simulink model "BLDC_OpenLoop_s32k144"  (Simulink 9.0)
settings: Solver=FixedStepDiscrete  StartTime=0.0  StopTime=10.0  FixedStep=0.1  RelTol=1e-3  EnableMultiTasking=on
model workspace (MAT data in the model file):
  ALIGN_TIME = Simulink.Parameter
  ALIGN_TIME.Value = 20
  ALIGN_TIME.Description = 'number of model fixed-step size steps.'
  ALIGN_TIME.DataType = 'uint16'
  ALIGN_TIME.Min = 0
  ALIGN_TIME.Max = 100
  ALIGN_TIME.Dimensions = [1 1]
  IDC_OVERCURRENT = Simulink.Parameter
  IDC_OVERCURRENT.Value = 4
  IDC_OVERCURRENT.DataType = 'single'
  IDC_OVERCURRENT.Min = 0
  IDC_OVERCURRENT.Max = 16
  IDC_OVERCURRENT.DocUnits = 'A'
  IDC_OVERCURRENT.Dimensions = [1 1]
  V0 = Simulink.Parameter
  V0.Value = 3
  V0.DataType = 'single'
  V0.Min = 0
  V0.Max = 12
  V0.DocUnits = 'V'
  V0.Dimensions = [1 1]
  VDC_OVERVOLTAGE = Simulink.Parameter
  VDC_OVERVOLTAGE.Value = 18
  VDC_OVERVOLTAGE.DataType = 'single'
  VDC_OVERVOLTAGE.Min = 0
  VDC_OVERVOLTAGE.Max = 18
  VDC_OVERVOLTAGE.DocUnits = 'V'
  VDC_OVERVOLTAGE.Dimensions = [1 1]
  VDC_UNDERVOLTAGE = Simulink.Parameter
  VDC_UNDERVOLTAGE.Value = 8
  VDC_UNDERVOLTAGE.DataType = 'single'
  VDC_UNDERVOLTAGE.Min = 0
  VDC_UNDERVOLTAGE.Max = 18
  VDC_UNDERVOLTAGE.DocUnits = 'V'
  VDC_UNDERVOLTAGE.Dimensions = [1 1]
InitFcn:
  | mbd_s32k_consistency_checks(bdroot(gcs));
undefined symbols (not defined in the file): External, LQFP, One, Shot, TRGMUX_PDB_TRIG
libraries: mbd_s32k1xx_ec_toolbox x40, simulink x8, mbd_msd_ec_toolbox x5, ammclib_bam_s32k14x x2
(part 1 of 2)
Description:
  | Open Loop BLDC example for S32K144 and DevKit MotorGD.
  | This Simulink model is designed to work with Linix 45ZWN24-40 Motor and validate
  | that the motor can be rotated with 6-step commutation method. The main scope of
  | the model is to validate the Hall sensors.
  | 
  | FEATURES:
  | - Voltage command is read via SW2 (CW direction) or SW3 (CCW direction)
  | - Read hall sensors in interrupt more for table commutation (used to drive the MOSFETs)
  | 
  | HW SETUP:
  | - Configure S32K144 board supply voltage: J107:2-3(over USB)
  | - Configure J9,J10 and J11 on MotorGD: 2-3 (mode BLDC)
  | - Rotate trimmer resistor R72 (placed Devkit-MotorGD) counter-clockwise at maximum
  | - Connect the motor phases to MotorGD J13 connector
  |   (i.e. Linix 45ZWN24-40: phA-white/phB-blue/phC-green)
  | - Connect the motor hall sensors to MotorGD JP1 connector
  |   (i.e. Linix 45ZWN24-40: Hall_A-white/Hall_B-blue/Hall_C-green)
  | - Power on the MotorGD via J7 connector with 12Vdc
  | - NOTE! Make sure the R168/R166 are placed and R167/R165 are removed
  | 
  | VALIDATION:
  | - After reset or power on, the Green LED shall be ON after ~5sec
  | - If the Vdc is present and SW2 or SW3 is pressed the Blue LED will be ON
  | - In case of a FAULT the Red LED will be ON
  | - The initial voltage command is set to 3V and can be changed from Simulink Model Wrks
  | - Open FreeMASTER project and connect to the target.
  | - Start by pressing the SW2 or SW3 to command the motor to spin in CW or CCW direction
  | - Press the SW2 or SW3 the modify the motor speed or use FreeMASTER UI panel
  | - Voltage and Current protections for Devkit MotorGD are enabled. If fault occurs the
  |   INVERTER is shut down and RED LED is ON
  | 
  | NOTE:
  | - In case of fault (RED LED is ON), the remove fault cause and press RESET button
  | 
  | Copyright (c) 2019 NXP
  | version 3.2.0
settings Model: Creator=NXP MBDT Team  LastModifiedBy=nxf40284  OrderedModelArguments=off
settings DataIOCC: ExternalInput=off  InitialState=off  LimitDataPoints=on  SaveOutput=off  SignalLogging=off  SaveTime=off
settings OptimizationCC: DefaultParameterBehavior=Inlined  UseFloatMulNetSlope=on  DefaultUnderspecifiedDataType=single  UseSpecifiedMinMax=on  EnhancedBackFolding=on  PassReuseOutputArgsAs=Individual arguments  ZeroExternalMemoryAtStartup=off  ZeroInternalMemoryAtStartup=off  NoFixptDivByZeroProtection=on  EfficientFloat2IntCast=on  LifeSpan=auto  OptimizeBlockOrder=speed  DifferentSizesBufferReuse=on
settings DebuggingCC: CheckSSInitialOutputMsg=off  SolverPrmCheckMsg=warning  InheritedTsInSrcMsg=none  MultiTaskDSMMsg=none  SingleTaskRateTransMsg=error  ParameterPrecisionLossMsg=none  ParameterTunabilityLossMsg=error  UnconnectedInputMsg=error  UnconnectedOutputMsg=error  UnconnectedLineMsg=error  AssertControl=DisableAll  AllowSymbolicDim=off  UnknownTsInhSupMsg=error  StateNameClashWarn=warning  ArithmeticOperatorsInVariantConditions=warning
settings HardwareCC: ProdLargestAtomicInteger=Long  ProdLargestAtomicFloat=Double  ProdIntDivRoundTo=Zero  ProdEndianess=LittleEndian  ProdHWDeviceType=ARM Compatible->ARM Cortex
settings ModelReferenceCC: PropagateSignalLabelsOutOfModel=on
settings SFSimCC: MATLABDynamicMemAlloc=off
settings RTWCC: SystemTargetFile=mbd_s32k.tlc  MakeCommand=mbd_s32k_make_rtw COPY_MDLREF_INCLUDES=0  TemplateMakefile=mbd_s32k.tmf  Description=Model Based Design Toolbox S32K1xx Code Generation Target  IncludeHyperlinkInReport=on
settings CodeAppCC: ForceParamTrailComments=on  IgnoreCustomStorageClasses=off  MaxIdLength=64  OperatorAnnotations=on  SimulinkDataObjDesc=on  SFDataObjDesc=on  InsertBlockDesc=on  StateflowObjectComments=off  InternalIdentifier=Classic
settings STFCustomTargetCC: TargetLangStandard=C99 (ISO)  MultiwordLength=256  CombineOutputUpdateFcns=on  ERTCustomFileBanners=on  SupportContinuousTime=off  SupportNonInlinedSFcns=off  RemoveResetFunc=on  MATLABClassNameForMDSCustomization=Simulink.SoftwareTarget.ERTCustomization  GRTInterface=off  SystemTargetFile=mbd_s32k.tlc
settings ERTTargetCC: TargetLangStandard=C99 (ISO)  ParMdlRefBuildCompliant=off  CompOptLevelCompliant=off  ConcurrentExecutionCompliant=off  ModelStepFunctionPrototypeControlCompliant=off  CPPClassGenCompliant=off  UseToolchainInfoCompliant=off  InlinedParameterPlacement=NonHierarchical  ERTSrcFileBannerTemplate=mbd_ert_code_template.cgt  ERTHdrFileBannerTemplate=mbd_ert_code_template.cgt  ERTDataSrcFileTemplate=mbd_ert_code_template.cgt  ERTDataHdrFileTemplate=mbd_ert_code_template.cgt  ERTCustomFileTemplate=example_file_process.tlc

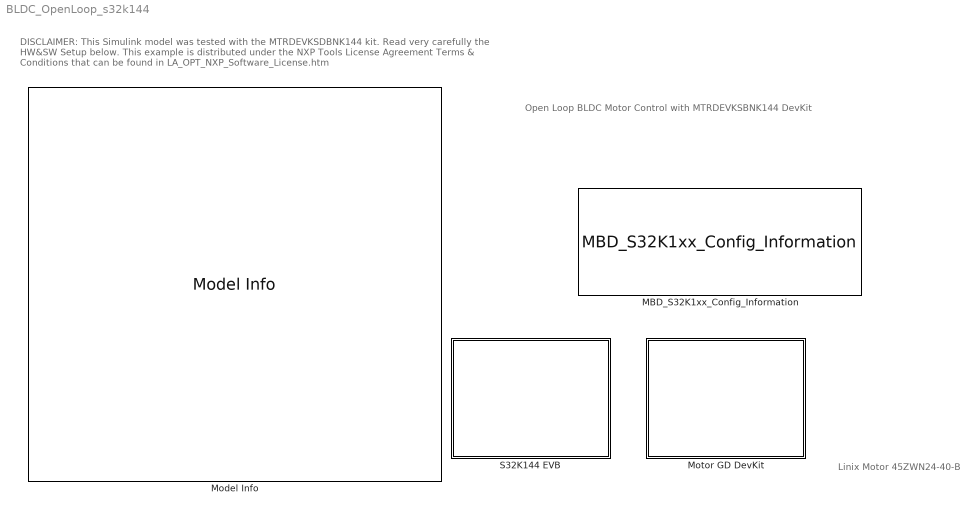
== system BLDC_OpenLoop_s32k144 ==
  note: Linix Motor 45ZWN24-40-B
  note: Open Loop BLDC Motor Control
      | with MTRDEVKSBNK144 DevKit
  note: DISCLAIMER: This Simulink model was tested with the MTRDEVKSDBNK144 kit. Read very carefully the HW&SW Setup below.
      | This example is distributed under the NXP Tools License Agreement Terms & Conditions that can be found in LA_OPT_NXP_Software_License.htm
  MBD_S32K1xx_Config_Information : mbd_s32k1xx_ec_toolbox/MBD_S32K1xx_Config_Information  mbdt_ver=0  disp_str=|  config_params=[]  mcu_target_name=S32K144  mcu_target_package=64-LQFP  mcu_target_sram_size=64KB  mcu_system_clock_freq=80  mcu_xtal_freq=External 8  mcu_steptick_timer=LPIT Channel 0  mcu_steptick_prio=10  ds_import_enable=on  target_compiler=GCC  target_memory=FLASH  gcc_target_compile_opts=-mcpu=cortex-m4 -mthumb -mfloat-abi=hard -mfpu=fpv4-sp-d16 -O1 -g -gstrict-dwarf  gcc_target_assemble_opts=-mcpu=cortex-m4 -mthumb -mfloat-abi=hard -mfpu=fpv4-sp-d16 -g  gcc_target_link_opts=-mcpu=cortex-m4 -mthumb -mfloat-abi=hard -mfpu=fpv4-sp-d16  gcc_target_default_lcf=on  gcc_target_user_lcf=S32K144_64_flash.ld  ghs_target_compile_opts=-cpu=cortexm4f -thumb -fpu=vfpv4_d16 -fsingle -Ogeneral -Wundef -Wimplicit-int -Wshadow -Wtrigraphs --no_commons --gnu_asm -gnu99 -gdwarf-2 -G  ghs_target_assemble_opts=-cpu=cortexm4f -fpu=vfpv4_d16  ghs_target_link_opts=-cpu=cortexm4f -thumb -fpu=vfpv4_d16  ghs_target_default_lcf=on  ghs_target_user_lcf=S32K144_64_flash.ld  iar_target_compile_opts=--cpu=Cortex-M4F --thumb --fpu=VFPv4_sp -Ol -e --debug --dlib_config normal  iar_target_assemble_opts=--cpu Cortex-M4F --thumb --fpu VFPv4_sp  iar_target_link_opts=--no_exceptions --vfe --inline  iar_target_default_lcf=on  iar_target_user_lcf=S32K144_64_flash.icf  pil_download_enable=off  rbl_download_enable=on  rbl_start_delay=5000  rbl_download_interface=OpenSDA  rbl_restart_request=off  rbl_com_port=Custom  rbl_com_port_custom=COM1  pil_download_rate=57600  pil_opensda_drive=Custom  pil_opensda_drive_custom=D  pil_uart_instance=1  pil_uart_rx=PTC6: [LPUART1_RX | Receive]  pil_uart_tx=PTC7: [LPUART1_TX | Transmit]  FTM_PWM_PcrCheckEnDis=on  FTM_Input_Edge_Inputs_PcrCheckEnDis=on  FTM_Dual_Edge_Inputs_PcrCheckEnDis=on  FTM_Quadrature_Inputs_PcrCheckEnDis=on  FTM_Hall_Sensor_Inputs_PcrCheckEnDis=on  LPTMR_PcrCheckEnDis=on  PIT_PcrCheckEnDis=on  RTC_PcrCheckEnDis=on  FlexCAN_PcrCheckEnDis=on  LIN_PcrCheckEnDis=on  FlexIO_PcrCheckEnDis=on  LPI2C_PcrCheckEnDis=on  LPSPI_PcrCheckEnDis=on  LPUART_PcrCheckEnDis=on  CMP_PcrCheckEnDis=on  GPIO_OutputPcrCheckEnDis=on  GPIO_InputPcrCheckEnDis=on  SBC_PcrCheckEnDis=on  AMMCLIB_PcrCheckEnDis=on  FM_PcrCheckEnDis=on  Profile_PcrCheckEnDis=on  ConfigParams_PcrCheckEnDis=on  ModelRef_PcrCheckEnDis=on  PDB0_PcrCheckEnDis=on  CSEc_PcrCheckEnDis=on  eDMA_PcrCheckEnDis=on  ADC_PcrCheckEnDis=on  WDOG_PcrCheckEnDis=on
      | Target : S32K144-64KB_SRAM
      | Package : 100-pin
      | System clock : 80 MHz
      | XTAL clock : External 8 MHz
      | Compiler : IAR
      | Target Type : FLASH
      | Download Code after build : off
      | Step Tick Interrupt Priority : 15
  Model Info : simulink/Model-Wide Utilities/Model Info  Frame=off  DisplayStringWithTags=|  HorizontalTextAlignment=Left  LeftAlignmentValue=0.02
      | Model Name: %<ModelName>
      | 
      | Description: %<Description>
  Motor GD DevKit : Subsystem
      mask Display: image('MotorGD.PNG');
  S32K144 EVB : Subsystem
      mask Display: image('S32K.PNG');

== system BLDC_OpenLoop_s32k144/Motor GD DevKit ==

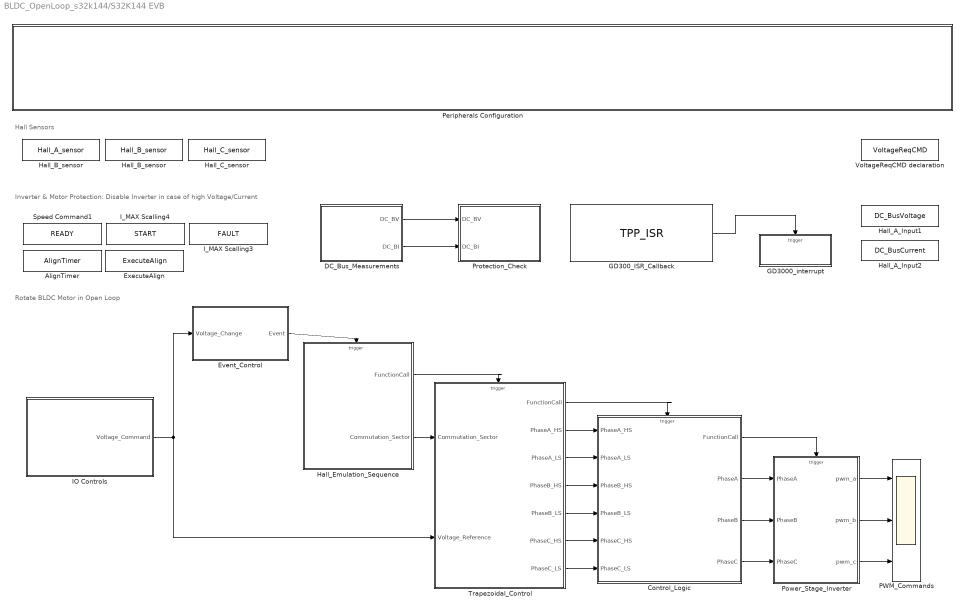
== system BLDC_OpenLoop_s32k144/S32K144 EVB ==
  note: Rotate BLDC Motor in Open Loop
  note: Inverter & Motor Protection: Disable Inverter in case of high Voltage/Current
  note: Hall Sensors
  AlignTimer : DataStoreMemory  DataStoreName=AlignTimer  ReadBeforeWriteMsg=warning  WriteAfterWriteMsg=warning  WriteAfterReadMsg=warning  ShowAdditionalParam=off  OutDataTypeStr=uint16
  Control_Logic : Subsystem
  DC_Bus_Measurements : Subsystem
  Event_Control : Subsystem  TreatAsAtomicUnit=on
      settings: RTWFcnNameOpts=Use subsystem name  RTWFileNameOpts=Use subsystem name
  ExecuteAlign : DataStoreMemory  DataStoreName=ExecuteAlign  ReadBeforeWriteMsg=warning  WriteAfterWriteMsg=warning  WriteAfterReadMsg=warning  InitialValue=1  ShowAdditionalParam=off  OutDataTypeStr=boolean
  GD3000_interrupt : Subsystem  TreatAsAtomicUnit=on
  "GD300_ISR_Callback " : mbd_msd_ec_toolbox/TPP/TPP_ISR  tppInstance=0
  Hall_A_Input1 : DataStoreMemory  DataStoreName=DC_BusVoltage  ReadBeforeWriteMsg=warning  WriteAfterWriteMsg=warning  WriteAfterReadMsg=warning  ShowAdditionalParam=off  OutDataTypeStr=single
  Hall_A_Input2 : DataStoreMemory  DataStoreName=DC_BusCurrent  ReadBeforeWriteMsg=warning  WriteAfterWriteMsg=warning  WriteAfterReadMsg=warning  ShowAdditionalParam=off  OutDataTypeStr=single
  Hall_B_sensor : DataStoreMemory  DataStoreName=Hall_A_sensor  ReadBeforeWriteMsg=warning  WriteAfterWriteMsg=warning  WriteAfterReadMsg=warning  ShowAdditionalParam=off  OutDataTypeStr=boolean
  "Hall_B_sensor " : DataStoreMemory  DataStoreName=Hall_B_sensor  ReadBeforeWriteMsg=warning  WriteAfterWriteMsg=warning  WriteAfterReadMsg=warning  ShowAdditionalParam=off  OutDataTypeStr=boolean
  "Hall_C_sensor " : DataStoreMemory  DataStoreName=Hall_C_sensor  ReadBeforeWriteMsg=warning  WriteAfterWriteMsg=warning  WriteAfterReadMsg=warning  ShowAdditionalParam=off  OutDataTypeStr=boolean
  Hall_Emulation_Sequence : Subsystem
      settings: PropExecContextOutsideSubsystem=on  RTWSystemCode=Nonreusable function  RTWFileNameOpts=Use subsystem name
  "IO Controls " : Subsystem
  I_MAX Scalling3 : DataStoreMemory  DataStoreName=FAULT  ReadBeforeWriteMsg=warning  WriteAfterWriteMsg=warning  WriteAfterReadMsg=warning  ShowAdditionalParam=off  OutDataTypeStr=boolean
  I_MAX Scalling4 : DataStoreMemory  DataStoreName=START  ReadBeforeWriteMsg=warning  WriteAfterWriteMsg=warning  WriteAfterReadMsg=warning  ShowAdditionalParam=off  OutDataTypeStr=boolean
  PWM_Commands : Scope  NumInputPorts=3
  Peripherals Configuration : Subsystem  Priority=1
  Power_Stage_Inverter : Subsystem  TreatAsAtomicUnit=on
      settings: RTWSystemCode=Nonreusable function
  Protection_Check : Subsystem
  Speed Command1 : DataStoreMemory  DataStoreName=READY  ReadBeforeWriteMsg=warning  WriteAfterWriteMsg=warning  WriteAfterReadMsg=warning  ShowAdditionalParam=off  OutMin=0  OutMax=1  OutDataTypeStr=boolean
  Trapezoidal_Control : Subsystem
      settings: RTWSystemCode=Nonreusable function  RTWFcnNameOpts=Use subsystem name
  VoltageReqCMD declaration : DataStoreMemory  Priority=0  DataStoreName=VoltageReqCMD  ReadBeforeWriteMsg=warning  WriteAfterWriteMsg=warning  WriteAfterReadMsg=warning  ShowAdditionalParam=off  OutMin=-12  OutMax=12  OutDataTypeStr=single
  wires:
  Trapezoidal_Control/5(PhaseB_LS) -> Control_Logic/4(PhaseB_LS)
  Trapezoidal_Control/1(FunctionCall) -> Control_Logic/Trigger
  Control_Logic/3(PhaseB) -> Power_Stage_Inverter/2(PhaseB)
  Control_Logic/4(PhaseC) -> Power_Stage_Inverter/3(PhaseC)
  Control_Logic/2(PhaseA) -> Power_Stage_Inverter/1(PhaseA)
  Trapezoidal_Control/6(PhaseC_HS) -> Control_Logic/5(PhaseC_HS)
  Trapezoidal_Control/3(PhaseA_LS) -> Control_Logic/2(PhaseA_LS)
  Control_Logic/1(FunctionCall) -> Power_Stage_Inverter/Trigger
  Trapezoidal_Control/2(PhaseA_HS) -> Control_Logic/1(PhaseA_HS)
  Trapezoidal_Control/7(PhaseC_LS) -> Control_Logic/6(PhaseC_LS)
  Trapezoidal_Control/4(PhaseB_HS) -> Control_Logic/3(PhaseB_HS)
  Power_Stage_Inverter/1(pwm_a) -> PWM_Commands/1
  Power_Stage_Inverter/2(pwm_b) -> PWM_Commands/2
  Power_Stage_Inverter/3(pwm_c) -> PWM_Commands/3
  Event_Control/1(Event) -> Hall_Emulation_Sequence/Trigger
  Hall_Emulation_Sequence/1(FunctionCall) -> Trapezoidal_Control/Trigger
  Hall_Emulation_Sequence/2(Commutation_Sector) -> Trapezoidal_Control/1(Commutation_Sector)
  "IO Controls "/1(Voltage_Command) -> Event_Control/1(Voltage_Change), Trapezoidal_Control/2(Voltage_Reference)
  DC_Bus_Measurements/1(DC_BV) -> Protection_Check/1(DC_BV)
  DC_Bus_Measurements/2(DC_BI) -> Protection_Check/2(DC_BI)
  "GD300_ISR_Callback "/1 -> GD3000_interrupt/Trigger

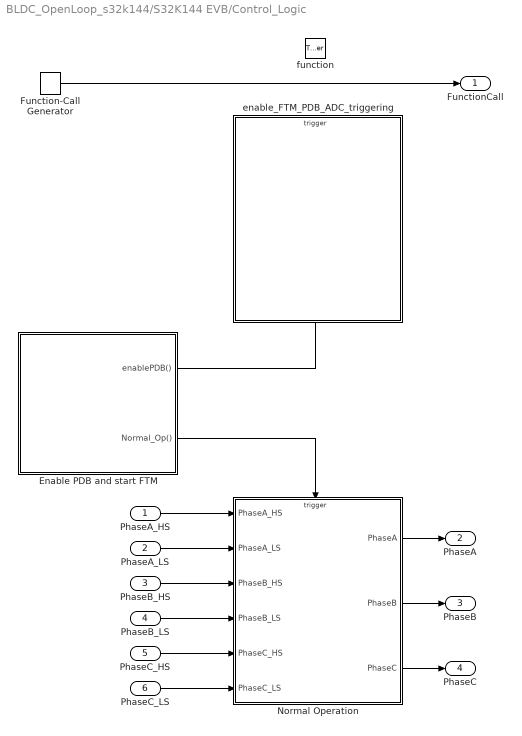
== system BLDC_OpenLoop_s32k144/S32K144 EVB/Control_Logic ==
  PhaseA_HS : Inport
  PhaseA_LS : Inport  Port=2
  PhaseB_HS : Inport  Port=3
  PhaseB_LS : Inport  Port=4
  PhaseC_HS : Inport  Port=5
  PhaseC_LS : Inport  Port=6
  function : TriggerPort  TriggerType=function-call  VariantControl=(inherit)
  Enable PDB and start FTM : Stateflow chart  TreatAsAtomicUnit=on
  Function-Call Generator : simulink/Ports & Subsystems/Function-Call Generator  sample_time=-1  numberOfIterations=1
  Normal Operation : Subsystem  TreatAsAtomicUnit=on
  enable_FTM_PDB_ADC_triggering : Subsystem  TreatAsAtomicUnit=on
      settings: RTWSystemCode=Inline
  FunctionCall : Outport
  PhaseA : Outport  Port=2
  PhaseB : Outport  Port=3
  PhaseC : Outport  Port=4
  wires:
  Enable PDB and start FTM/2(Normal_Op()) -> Normal Operation/Trigger
  Enable PDB and start FTM/1(enablePDB()) -> enable_FTM_PDB_ADC_triggering/Trigger
  Function-Call Generator/1 -> FunctionCall/1
  PhaseB_HS/1 -> Normal Operation/3(PhaseB_HS)
  PhaseB_LS/1 -> Normal Operation/4(PhaseB_LS)
  PhaseA_LS/1 -> Normal Operation/2(PhaseA_LS)
  PhaseC_HS/1 -> Normal Operation/5(PhaseC_HS)
  PhaseA_HS/1 -> Normal Operation/1(PhaseA_HS)
  PhaseC_LS/1 -> Normal Operation/6(PhaseC_LS)
  Normal Operation/2(PhaseB) -> PhaseB/1
  Normal Operation/3(PhaseC) -> PhaseC/1
  Normal Operation/1(PhaseA) -> PhaseA/1

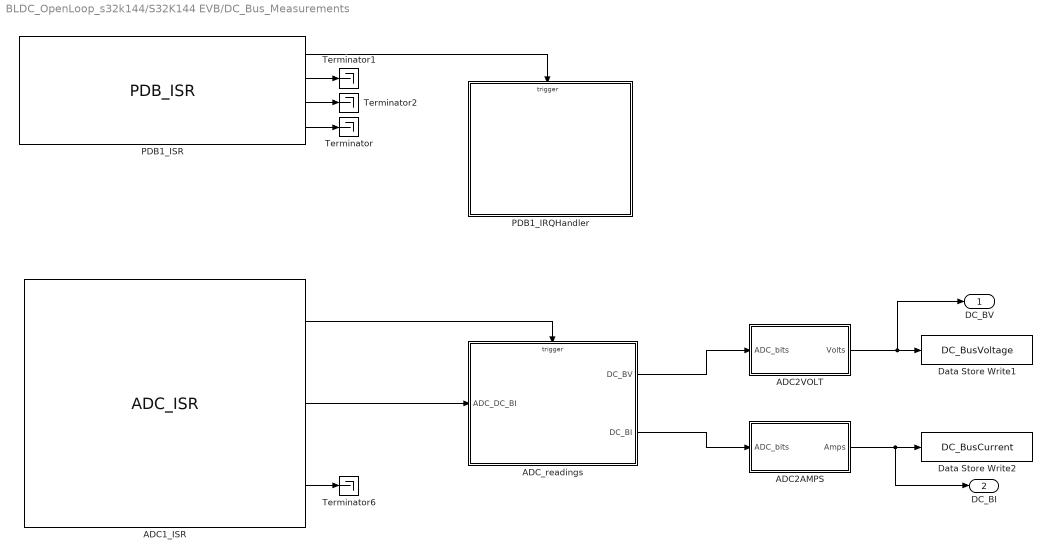
== system BLDC_OpenLoop_s32k144/S32K144 EVB/DC_Bus_Measurements ==
  ADC1_ISR : mbd_s32k1xx_ec_toolbox/Motor Control Blocks/ADC Blocks/ADC_ISR  instance=1  pri=1  sc1n=B
  ADC2AMPS : Subsystem
  ADC2VOLT : Subsystem
  ADC_readings : Subsystem  TreatAsAtomicUnit=on
      settings: RTWSystemCode=Nonreusable function
  Data Store Write1 : DataStoreWrite  DataStoreName=DC_BusVoltage
  Data Store Write2 : DataStoreWrite  DataStoreName=DC_BusCurrent
  PDB1_IRQHandler : Subsystem  TreatAsAtomicUnit=on
      settings: RTWSystemCode=Nonreusable function
  PDB1_ISR : mbd_s32k1xx_ec_toolbox/Motor Control Blocks/PDB Blocks/PDB_ISR  pdbModule=1  prioInterrupt=2  regScPdbie=on  regScPdbeie=off  regIdlyIdly=4999
  Terminator{,1..2,6} (4 alike) : Terminator
  DC_BV : Outport
  DC_BI : Outport  Port=2
  wires:
  ADC2VOLT/1(Volts) -> DC_BV/1, Data Store Write1/1
  ADC_readings/1(DC_BV) -> ADC2VOLT/1(ADC_bits)
  ADC2AMPS/1(Amps) -> DC_BI/1, Data Store Write2/1
  ADC_readings/2(DC_BI) -> ADC2AMPS/1(ADC_bits)
  PDB1_ISR/1 -> PDB1_IRQHandler/Trigger
  PDB1_ISR/4 -> Terminator/1
  PDB1_ISR/2 -> Terminator1/1
  PDB1_ISR/3 -> Terminator2/1
  ADC1_ISR/1 -> ADC_readings/Trigger
  ADC1_ISR/3 -> Terminator6/1
  ADC1_ISR/2 -> ADC_readings/1(ADC_DC_BI)

== system BLDC_OpenLoop_s32k144/S32K144 EVB/Event_Control ==
  Voltage_Change : Inport
  ControlEventLogic : Subsystem  Priority=3
  ControlPollingLogic : Stateflow chart  Priority=2  TreatAsAtomicUnit=on
  HallSensorInit : Subsystem
      settings: RTWFcnNameOpts=Use subsystem name  RTWFileNameOpts=Use subsystem name
  Init : Stateflow chart  Priority=1  TreatAsAtomicUnit=on
  Mux1 : Mux  Inputs=3
  Event : Outport
  wires:
  Mux1/1 -> Event/1
  Voltage_Change/1 -> ControlPollingLogic/1(VoltageChange)
  Init/1(Init()) -> HallSensorInit/Trigger
  ControlEventLogic/1(HallStateChange) -> Mux1/3
  ControlPollingLogic/1(Trigger()) -> Mux1/2
  HallSensorInit/1(Call) -> Mux1/1

== system BLDC_OpenLoop_s32k144/S32K144 EVB/GD3000_interrupt ==
  function : TriggerPort  TriggerType=function-call  VariantControl=Variant
  FAULT_write : DataStoreWrite  DataStoreName=FAULT
  FTM_PWM_Disable_Enable : mbd_s32k1xx_ec_toolbox/Motor Control Blocks/FTM Blocks/FTM_PWM_Disable_Enable  ftmModule=3  action=Disable
  NOK : Constant  OutDataTypeStr=boolean
  TPP_Functional_Mode : mbd_msd_ec_toolbox/TPP/TPP_Functional_Mode  tppInstance=0  action=Sleep
  wires:
  NOK/1 -> FAULT_write/1

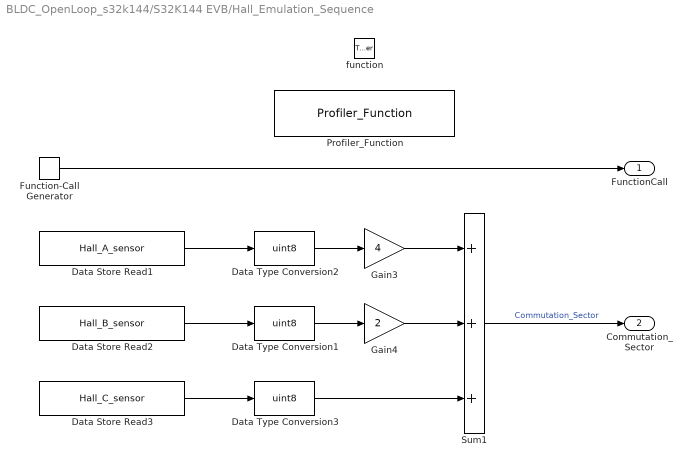
== system BLDC_OpenLoop_s32k144/S32K144 EVB/Hall_Emulation_Sequence ==
  function : TriggerPort  TriggerType=function-call  VariantControl=Variant
  Data Store Read1 : DataStoreRead  DataStoreName=Hall_A_sensor
  Data Store Read2 : DataStoreRead  DataStoreName=Hall_B_sensor
  Data Store Read3 : DataStoreRead  DataStoreName=Hall_C_sensor
  Data Type Conversion1 : DataTypeConversion  OutDataTypeStr=uint8
  Data Type Conversion2 : DataTypeConversion  OutDataTypeStr=uint8
  Data Type Conversion3 : DataTypeConversion  OutDataTypeStr=uint8
  Function-Call Generator : simulink/Ports & Subsystems/Function-Call Generator  sample_time=-1  numberOfIterations=1
  Gain3 : Gain  Gain=4  OutDataTypeStr=uint8  ParamDataTypeStr=Inherit: Same as input
  Gain4 : Gain  Gain=2  OutDataTypeStr=uint8  ParamDataTypeStr=Inherit: Same as input
  Profiler_Function : mbd_s32k1xx_ec_toolbox/Utility Blocks/Profiler_Function  profile_indx=0
  Sum1 : Sum  Inputs=+++  AccumDataTypeStr=uint8
  FunctionCall : Outport
  Commutation_Sector : Outport  Port=2  OutDataTypeStr=uint8
  wires:
  Function-Call Generator/1 -> FunctionCall/1
  Gain3/1 -> Sum1/1
  Gain4/1 -> Sum1/2
  Data Type Conversion2/1 -> Gain3/1
  Data Type Conversion1/1 -> Gain4/1
  Data Type Conversion3/1 -> Sum1/3
  Data Store Read1/1 -> Data Type Conversion2/1
  Data Store Read2/1 -> Data Type Conversion1/1
  Data Store Read3/1 -> Data Type Conversion3/1
  Sum1/1 -> Commutation_Sector/1  "Commutation_Sector"

== system BLDC_OpenLoop_s32k144/S32K144 EVB/IO Controls  ==
  note: RUN STATE
  note: SYSTEM STATE
  If Action Subsystem : Subsystem  TreatAsAtomicUnit=on
  If1 : If  IfExpression=(u1 == 1)  ShowElse=off
  If2 : If  IfExpression=(u1 == 1)  ShowElse=off
  SpeedCmd1 : DataStoreRead  DataStoreName=START
  SpeedCmd2 : DataStoreRead  DataStoreName=FAULT
  SpeedCmd3 : DataStoreRead  DataStoreName=START
  SpeedCmd4 : DataStoreRead  DataStoreName=READY
  Subsystem : Subsystem
  Voltage_Command : Outport
  wires:
  SpeedCmd1/1 -> If1/1
  If1/1 -> If Action Subsystem/Action
  If Action Subsystem/1(Voltage_Command) -> Voltage_Command/1
  SpeedCmd3/1 -> Subsystem/1(START)
  SpeedCmd2/1 -> Subsystem/2(FAULT)
  SpeedCmd4/1 -> If2/1
  If2/1 -> Subsystem/Action

== system BLDC_OpenLoop_s32k144/S32K144 EVB/Peripherals Configuration ==
  ADC1_IRQ : mbd_s32k1xx_ec_toolbox/Motor Control Blocks/ADC Blocks/ADC_Start  Priority=3  instance=1  adc_r=B  adc_chan=PTD4: [ADC1_SE6 | ADC Single Ended Input]  aien=on  mcuTargetUpdate=on
  ADC_Config : mbd_s32k1xx_ec_toolbox/Motor Control Blocks/ADC Blocks/ADC_Config  Priority=2  instance=1  mode=12-bit conversion  smplts=2  adiclk=alternate clock 1  adiv=input clock  show_adv_opts=on  pretrgsel=PDB pre-trigger  swpretrg=Disabled  adtrg=hardware  trgsel=PDB output  refsel=Vrefh and Vrefl  supply_monitoring=off  acfe=off  acfgt=off  acren=off  cv1=0  cv2=0  adco=off  avge=off  avgs=16 samples
  Digital_Input_ISR_Enable_HALL_A : mbd_s32k1xx_ec_toolbox/GPIO Blocks/Digital_Input_ISR_Enable_Disable  gpio_pin=PTD11: [PTD11 | Port D I/O]  irqc=on either-edge
  Digital_Input_ISR_Enable_HALL_B : mbd_s32k1xx_ec_toolbox/GPIO Blocks/Digital_Input_ISR_Enable_Disable  gpio_pin=PTD10: [PTD10 | Port D I/O]  irqc=on either-edge
  Digital_Input_ISR_Enable_HALL_C : mbd_s32k1xx_ec_toolbox/GPIO Blocks/Digital_Input_ISR_Enable_Disable  gpio_pin=PTA1: [PTA1 | Port A I/O]  irqc=on either-edge
  FreeMaster_Config : mbd_s32k1xx_ec_toolbox/Utility Blocks/FreeMaster_Config  interface=LPUART1  baudrate=115200  rxd=PTC6: [LPUART1_RX | Receive]  txd=PTC7: [LPUART1_TX | Transmit]  mode=Short Interrupt  isr_prio=5  show_adv_opts=on  use_scope=on  max_scope_vars=8  use_recorder=on  max_rec_vars=8  rec_buff_size=2048  rec_timebase=1 milliseconds  comm_buffer_size_auto=on  comm_buffer_size=255  comm_rqueue_size_default=on  comm_rqueue_size=32
  GD3000_Config : mbd_msd_ec_toolbox/TPP/TPP_Config  Priority=1  tppInstance=0  desatMode=on  fullonMode=off  lockMode=off  overtempEvent=on  phaseEvent=off  desatEvent=off  framingEvent=on  vlsEvent=on  writeErrEvent=on  overcurrentEvent=on  resetEvent=on  mcuTppIntEn=off  prioInt=15  tppDeadtime=500  initTppNow=on  tppSpiInst=0  tppPwmModule=Please add FTM block to workspace  tppPair0_1=on  tppPair2_3=on  tppPair4_5=on  tppPair6_7=off  tppFirstChHS=on  tppEn1Pin=PTA2: [PTA2 | Port A I/O]  tppEn2Pin=PTA2: [PTA2 | Port A I/O]  tppRstPin=PTA3: [PTA3 | Port A I/O]  tppCsPin=PTB5: [PTB5 | Port B I/O]  tppIntPin=PTE10: [PTE10 | Port E I/O]
  "LPSPI_Config " : mbd_s32k1xx_ec_toolbox/Communication Blocks/SPI Blocks/LPSPI_Config   InstanceNumber=0  Role=Master  BaudRate=2000000  ShowAdvanced=on  sin=PTB3: [LPSPI0_SIN | LPSPI Serial Data Input]  sout=PTB4: [LPSPI0_SOUT | LPSPI Serial Data Output]  sck=PTB2: [LPSPI0_SCK | LPSPI Serial Clock I/O]  pcs0=None  pcs1=PTB5: [LPSPI0_PCS1 | Peripheral Chip Select 1]  pcs2=None  pcs3=None  CPHA=1  CPOL=0  BitOrder=MSB first  TransferSize=8  WhichPCS=0  PCSPol=ActiveLow  ContinuousTransfer=off
  PDB_Config : mbd_s32k1xx_ec_toolbox/Motor Control Blocks/PDB Blocks/PDB_Config  Priority=1  pdbModule=1  regScCont=One-Shot  regScTrgsel=External (TRGMUX_PDB_TRIG)  trgMuxSel=FTM3 Initialize Trigger  trgMuxSelPin=PTB5: [TRGMUX_IN0 | Trigger Mux Input]  regModModulus=5000  regScPrescaler=1  regScMult=1  regPoenPoen0=off  regPo0DlyDly1=0  regPo0DlyDly2=1000  enable_pdb_init=off  show_adv_opts=on  regCh0C1En0=on  regCh0C1En1=on  regCh0C1En2=off  regCh0C1En3=off  regCh0C1En4=off  regCh0C1En5=off  regCh0C1En6=off  regCh0C1En7=off  regCh0C1Bb0=off  regCh0C1Bb1=off  regCh0C1Bb2=off  regCh0C1Bb3=off  regCh0C1Bb4=off  regCh0C1Bb5=off  regCh0C1Bb6=off  regCh0C1Bb7=off  regCh0C1Tos0=Pre-trigger is in delay mode  regCh0C1Tos1=Pre-trigger is in delay mode  regCh0C1Tos2=Pre-trigger is in delay mode  regCh0C1Tos3=Pre-trigger is in delay mode  regCh0C1Tos4=Pre-trigger is in delay mode  regCh0C1Tos5=Pre-trigger is in delay mode  regCh0C1Tos6=Pre-trigger is in delay mode  regCh0C1Tos7=Pre-trigger is in delay mode  regCh0DlyDly0=0  regCh0DlyDly1=200  regCh0DlyDly2=0  regCh0DlyDly3=0  regCh0DlyDly4=0  regCh0DlyDly5=0  regCh0DlyDly6=0  regCh0DlyDly7=0  regCh1C1En0=off  regCh1C1En1=off  regCh1C1En2=off  regCh1C1En3=off  regCh1C1En4=off  regCh1C1En5=off  regCh1C1En6=off  regCh1C1En7=off  regCh1C1Bb0=off  regCh1C1Bb1=off  regCh1C1Bb2=off  regCh1C1Bb3=off  regCh1C1Bb4=off  regCh1C1Bb5=off  regCh1C1Bb6=off  regCh1C1Bb7=off  regCh1C1Tos0=Pre-trigger is in delay mode  regCh1C1Tos1=Pre-trigger is in delay mode  regCh1C1Tos2=Pre-trigger is in delay mode  regCh1C1Tos3=Pre-trigger is in delay mode  regCh1C1Tos4=Pre-trigger is in delay mode  regCh1C1Tos5=Pre-trigger is in delay mode  regCh1C1Tos6=Pre-trigger is in delay mode  regCh1C1Tos7=Pre-trigger is in delay mode  regCh1DlyDly0=100  regCh1DlyDly1=200  regCh1DlyDly2=300  regCh1DlyDly3=400  regCh1DlyDly4=500  regCh1DlyDly5=600  regCh1DlyDly6=700  regCh1DlyDly7=800

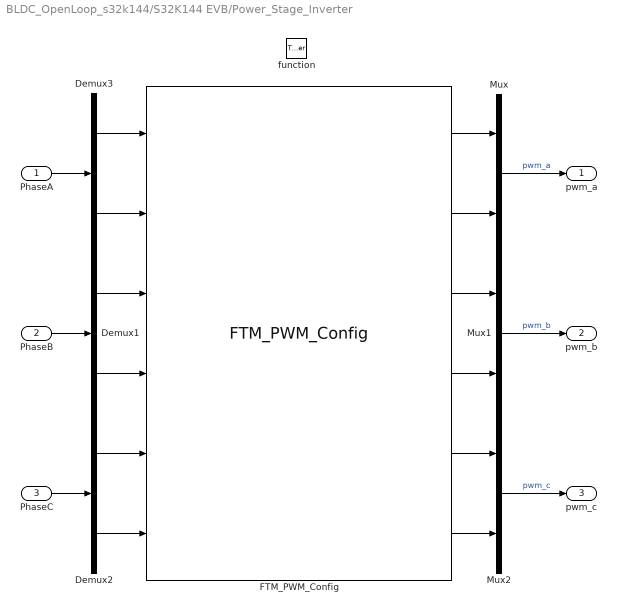
== system BLDC_OpenLoop_s32k144/S32K144 EVB/Power_Stage_Inverter ==
  PhaseA : Inport
  PhaseB : Inport  Port=2
  PhaseC : Inport  Port=3
  function : TriggerPort  TriggerType=function-call  VariantControl=Variant
  Demux1 : Demux  Outputs=2
  Demux2 : Demux  Outputs=2
  Demux3 : Demux  Outputs=2
  FTM_PWM_Config : mbd_s32k1xx_ec_toolbox/Motor Control Blocks/FTM Blocks/FTM_PWM_Config  ftmModule=3  ftmMode=Center-Aligned PWM  ftmSourceClock=80 MHz  swcontrol_enable=off  chan0En=on  chan0Type=Independent  chan2En=on  chan2Type=Independent  chan4En=on  chan4Type=Independent  chan6En=off  chan6Type=Independent  ftmPwmUnits=Hz  outFrequency=20000  ftmPeriod=4000  ftmPrescaler=Divide by 1  deadtimeUnits=Nanoseconds  deadtimeNs=0  deadtimeTicks=0  deadtimePrescaler=Divide by 1  dutyCycleCh0=0  dutyCycleCh1=0  dutyCycleCh2=0  dutyCycleCh3=0  dutyCycleCh4=0  dutyCycleCh5=0  dutyCycleCh6=0.25  dutyCycleCh7=0.25  dutyCycleSim=on  startAfterInit=off  showAdvOpt=on  pinFtmCh0=PTB8: [FTM3_CH0 | FTM Channel]  pinFtmCh1=PTB9: [FTM3_CH1 | FTM Channel]  pinPolCh0=Active Low  pinPolCh1=Active High  outputComplem0=Main duplicated  outputLevel0=Low  outputLevel1=Low  pinFtmCh2=PTB10: [FTM3_CH2 | FTM Channel]  pinFtmCh3=PTB11: [FTM3_CH3 | FTM Channel]  pinPolCh2=Active Low  pinPolCh3=Active High  outputComplem2=Main duplicated  outputLevel2=Low  outputLevel3=Low  pinFtmCh4=PTC10: [FTM3_CH4 | FTM Channel]  pinFtmCh5=PTC11: [FTM3_CH5 | FTM Channel]  pinPolCh4=Active Low  pinPolCh5=Active High  outputComplem4=Main duplicated  outputLevel4=Low  outputLevel5=Low  pinFtmCh6=PTC12: [FTM3_CH6 | FTM Channel]  pinFtmCh7=None  pinPolCh6=Active Low  pinPolCh7=Active Low  outputComplem6=Main duplicated  outputLevel6=Low  outputLevel7=Low  initTrigger=off  chTrigger0=off  chTrigger1=off  chTrigger2=off  chTrigger3=off  chTrigger4=off  chTrigger5=off  chTrigger6=off  chTrigger7=off  mcuTargetUpdate=on  pwmSyncTrg=Software trigger  pwmSyncHwRouting=TRGMUX_FTM7  pwmSyncTrg0=off  pwmSyncTrg1=off  pwmSyncTrg2=off  pwmSyncAutoClear=off  pwmSyncMinLoad=off  pwmSyncMaxLoad=on  pwmSyncInvert=PWM Syncronization  pwmSyncOutControl=PWM Syncronization  pwmSyncOutMask=PWM Syncronization  pwmSyncCounterInitial=PWM Syncronization  pwmSyncPoints=Wait Loading Points  reloadEnable=off  reloadPriority=15  reloadHalfCycle=off  reloadHCR=0  reloadFrequency=0  chnMatch0=off  chnMatch1=off  chnMatch2=off  chnMatch3=off  chnMatch4=off  chnMatch5=off  chnMatch6=off  chnMatch7=off  pwmFaultProtection=off  pwmFaultInterrupt=off  pwmFaultClearing=Fault control disabled  pwmFaultPinState=Safe Value  pwmFaultFilterValue=0  pwmFaultPriority=15  fault_disen_0=off  fault_filter_0=off  fault_polarity_0=Active High  fault_disen_1=off  fault_filter_1=off  fault_polarity_1=Active high  fault_disen_2=off  fault_filter_2=off  fault_polarity_2=Active high  fault_disen_3=off  fault_filter_3=off  fault_polarity_3=Active high  fault_pin_0=None  fault_pin_1=None  fault_pin_2=None  fault_pin_3=None
  Mux : Mux  Inputs=2
  Mux1 : Mux  Inputs=2
  Mux2 : Mux  Inputs=2
  pwm_a : Outport
  pwm_b : Outport  Port=2
  pwm_c : Outport  Port=3
  wires:
  PhaseC/1 -> Demux2/1
  FTM_PWM_Config/1 -> Mux/1
  FTM_PWM_Config/2 -> Mux/2
  Mux/1 -> pwm_a/1  "pwm_a"
  Mux1/1 -> pwm_b/1  "pwm_b"
  FTM_PWM_Config/4 -> Mux1/2
  FTM_PWM_Config/3 -> Mux1/1
  Mux2/1 -> pwm_c/1  "pwm_c"
  FTM_PWM_Config/5 -> Mux2/1
  FTM_PWM_Config/6 -> Mux2/2
  Demux2/1 -> FTM_PWM_Config/5
  Demux2/2 -> FTM_PWM_Config/6
  Demux3/1 -> FTM_PWM_Config/1
  Demux3/2 -> FTM_PWM_Config/2
  Demux1/1 -> FTM_PWM_Config/3
  Demux1/2 -> FTM_PWM_Config/4
  PhaseB/1 -> Demux1/1
  PhaseA/1 -> Demux3/1

== system BLDC_OpenLoop_s32k144/S32K144 EVB/Protection_Check ==
  DC_BV : Inport
  DC_BI : Inport  Port=2
  " ALIGN_TMR" : DataStoreRead  DataStoreName=ExecuteAlign
  Abs : Abs
  Abs1 : Abs
  GDFLIB_FilterMA_FLT : ammclib_bam_s32k14x/GDFLIB/bam_flt/GDFLIB_FilterMA_FLT  fltLambda=10
  GDFLIB_FilterMA_FLT1 : ammclib_bam_s32k14x/GDFLIB/bam_flt/GDFLIB_FilterMA_FLT  fltLambda=10
  If1 : If  NumInputs=2  IfExpression=(u1 == 1) & (u2 == 0)  ShowElse=off
  SpeedCmd1 : DataStoreRead  DataStoreName=START
  Subsystem : Subsystem
  wires:
  DC_BV/1 -> Abs1/1
  DC_BI/1 -> Abs/1
  Abs1/1 -> GDFLIB_FilterMA_FLT/1
  Abs/1 -> GDFLIB_FilterMA_FLT1/1
  If1/1 -> Subsystem/Action
  SpeedCmd1/1 -> If1/1
  GDFLIB_FilterMA_FLT/1 -> Subsystem/1(In1)
  GDFLIB_FilterMA_FLT1/1 -> Subsystem/2(In2)
  " ALIGN_TMR"/1 -> If1/2

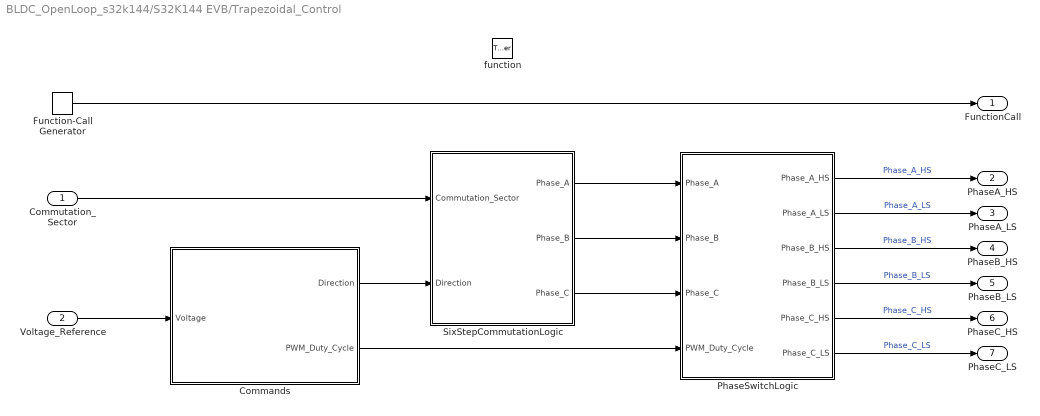
== system BLDC_OpenLoop_s32k144/S32K144 EVB/Trapezoidal_Control ==
  Commutation_Sector : Inport
  Voltage_Reference : Inport  Port=2
  function : TriggerPort  TriggerType=function-call  VariantControl=Variant
  Commands : Subsystem
  Function-Call Generator : simulink/Ports & Subsystems/Function-Call Generator  sample_time=-1  numberOfIterations=1
  PhaseSwitchLogic : Stateflow chart  TreatAsAtomicUnit=on
  SixStepCommutationLogic : Subsystem
  FunctionCall : Outport
  PhaseA_HS : Outport  Port=2
  PhaseA_LS : Outport  Port=3
  PhaseB_HS : Outport  Port=4
  PhaseB_LS : Outport  Port=5
  PhaseC_HS : Outport  Port=6
  PhaseC_LS : Outport  Port=7
  wires:
  Function-Call Generator/1 -> FunctionCall/1
  PhaseSwitchLogic/1(Phase_A_HS) -> PhaseA_HS/1  "Phase_A_HS"
  PhaseSwitchLogic/2(Phase_A_LS) -> PhaseA_LS/1  "Phase_A_LS"
  PhaseSwitchLogic/3(Phase_B_HS) -> PhaseB_HS/1  "Phase_B_HS"
  PhaseSwitchLogic/4(Phase_B_LS) -> PhaseB_LS/1  "Phase_B_LS"
  PhaseSwitchLogic/5(Phase_C_HS) -> PhaseC_HS/1  "Phase_C_HS"
  PhaseSwitchLogic/6(Phase_C_LS) -> PhaseC_LS/1  "Phase_C_LS"
  Commutation_Sector/1 -> SixStepCommutationLogic/1(Commutation_Sector)
  SixStepCommutationLogic/1(Phase_A) -> PhaseSwitchLogic/1(Phase_A)
  SixStepCommutationLogic/2(Phase_B) -> PhaseSwitchLogic/2(Phase_B)
  SixStepCommutationLogic/3(Phase_C) -> PhaseSwitchLogic/3(Phase_C)
  Voltage_Reference/1 -> Commands/1(Voltage)
  Commands/1(Direction) -> SixStepCommutationLogic/2(Direction)
  Commands/2(PWM_Duty_Cycle) -> PhaseSwitchLogic/4(PWM_Duty_Cycle)

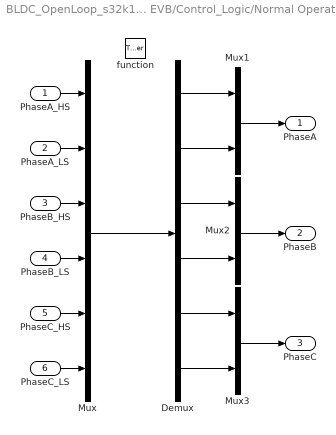
== system BLDC_OpenLoop_s32k144/S32K144 EVB/Control_Logic/Normal Operation ==
  PhaseA_HS : Inport
  PhaseA_LS : Inport  Port=2
  PhaseB_HS : Inport  Port=3
  PhaseB_LS : Inport  Port=4
  PhaseC_HS : Inport  Port=5
  PhaseC_LS : Inport  Port=6
  function : TriggerPort  TriggerType=function-call  VariantControl=(inherit)
  Demux : Demux  Outputs=6
  Mux : Mux  Inputs=6
  Mux1 : Mux  Inputs=2
  Mux2 : Mux  Inputs=2
  Mux3 : Mux  Inputs=2
  PhaseA : Outport
  PhaseB : Outport  Port=2
  PhaseC : Outport  Port=3
  wires:
  Mux/1 -> Demux/1
  Demux/4 -> Mux2/2
  Demux/2 -> Mux1/2
  Demux/3 -> Mux2/1
  Demux/5 -> Mux3/1
  Demux/1 -> Mux1/1
  Mux2/1 -> PhaseB/1
  Mux1/1 -> PhaseA/1
  Demux/6 -> Mux3/2
  Mux3/1 -> PhaseC/1
  PhaseA_HS/1 -> Mux/1
  PhaseA_LS/1 -> Mux/2
  PhaseB_HS/1 -> Mux/3
  PhaseB_LS/1 -> Mux/4
  PhaseC_HS/1 -> Mux/5
  PhaseC_LS/1 -> Mux/6

== system BLDC_OpenLoop_s32k144/S32K144 EVB/Control_Logic/enable_FTM_PDB_ADC_triggering ==
  function : TriggerPort  TriggerType=function-call  VariantControl=(inherit)
  Custom code to reload the PDB value : Subsystem  Priority=4  mask(System Outputs){ShowInLibBrowser=0}
      mask prompts: ShowInLibBrowser "Simulink:masks:CustCodeMaskParam1_MP"
      settings: CopyFcn=cccopyfcn(gcb)  OpenFcn=ccopenfcn('System Outputs Function')
      mask Help: eval('feval(''rtwprivate'',''rtwhelpview'',''rtw_sys_outputs_block'')');
      mask Display: disp('System\nOutputs');
  FTM3_PWM_Enable : mbd_s32k1xx_ec_toolbox/Motor Control Blocks/FTM Blocks/FTM_PWM_Disable_Enable  Priority=1  ftmModule=3  action=Enable
  FTM_Init_Trigger_Disable_Enable : mbd_s32k1xx_ec_toolbox/Motor Control Blocks/FTM Blocks/FTM_Init_Trigger_Disable_Enable  Priority=2  ftmModule=3  action=Enable
  ON : Constant  Priority=1  OutDataTypeStr=boolean
  PDB1_Enable : mbd_s32k1xx_ec_toolbox/Motor Control Blocks/PDB Blocks/PDB_Enable  Priority=3  pdbModule=1  pdbAction=Enable
  "SpeedCmd " : DataStoreWrite  DataStoreName=READY
  "TPP_ISR_Enable_Disable " : mbd_msd_ec_toolbox/TPP/TPP_ISR_Enable_Disable  Priority=4  tppInstance=0  mcuTppIntEn=on  prioInt=15
  wires:
  ON/1 -> "SpeedCmd "/1

== system BLDC_OpenLoop_s32k144/S32K144 EVB/DC_Bus_Measurements/ADC2AMPS ==
  ADC_bits : Inport
  Current_offset : Constant  Value=0.2  OutDataTypeStr=Inherit: Inherit via back propagation
  Sum : Sum  Inputs=+-  OutDataTypeStr=single
  Sum1 : Sum  Inputs=+-  OutDataTypeStr=single
  bits2amps : Gain  Gain=25/4095  OutDataTypeStr=single
  offset : Constant  Value=2048  OutDataTypeStr=uint32
  Amps : Outport
  wires:
  Sum/1 -> bits2amps/1
  offset/1 -> Sum/2
  ADC_bits/1 -> Sum/1
  Sum1/1 -> Amps/1
  bits2amps/1 -> Sum1/1
  Current_offset/1 -> Sum1/2

== system BLDC_OpenLoop_s32k144/S32K144 EVB/DC_Bus_Measurements/ADC2VOLT ==
  ADC_bits : Inport
  bits2volts : Gain  Gain=45/4095  OutDataTypeStr=single
  Volts : Outport
  wires:
  bits2volts/1 -> Volts/1
  ADC_bits/1 -> bits2volts/1

== system BLDC_OpenLoop_s32k144/S32K144 EVB/DC_Bus_Measurements/ADC_readings ==
  ADC_DC_BI : Inport  Priority=3
  function : TriggerPort  TriggerType=function-call  VariantControl=Variant
  FTM_Init_Trigger_Disable : mbd_s32k1xx_ec_toolbox/Motor Control Blocks/FTM Blocks/FTM_Init_Trigger_Disable_Enable  Priority=2  ftmModule=3  action=Disable
  Read_DC_Voltage : mbd_s32k1xx_ec_toolbox/Motor Control Blocks/ADC Blocks/ADC_Start  Priority=4  instance=1  adc_r=A  adc_chan=PTB12: [ADC1_SE7 | ADC Single Ended Input]  aien=off  mcuTargetUpdate=on
  DC_BV : Outport
  DC_BI : Outport  Port=2
  wires:
  Read_DC_Voltage/1 -> DC_BV/1
  ADC_DC_BI/1 -> DC_BI/1

== system BLDC_OpenLoop_s32k144/S32K144 EVB/DC_Bus_Measurements/PDB1_IRQHandler ==
  function : TriggerPort  TriggerType=function-call  VariantControl=(inherit)
  FTM_Init_Trigger_Enable : mbd_s32k1xx_ec_toolbox/Motor Control Blocks/FTM Blocks/FTM_Init_Trigger_Disable_Enable  ftmModule=3  action=Enable

== system BLDC_OpenLoop_s32k144/S32K144 EVB/Event_Control/ControlEventLogic ==
  Digital_Input_ISR_HALL_A : mbd_s32k1xx_ec_toolbox/GPIO Blocks/Digital_Input_ISR  gpio_pin=PTD11: [PTD11 | Port D I/O]  irqc=on either-edge  prio=5
  Digital_Input_ISR_HALL_B : mbd_s32k1xx_ec_toolbox/GPIO Blocks/Digital_Input_ISR  gpio_pin=PTD10: [PTD10 | Port D I/O]  irqc=on either-edge  prio=5
  Digital_Input_ISR_HALL_C : mbd_s32k1xx_ec_toolbox/GPIO Blocks/Digital_Input_ISR  gpio_pin=PTA1: [PTA1 | Port A I/O]  irqc=on either-edge  prio=5
  Mux2 : Mux  Inputs=3
  Toggle_HallA : Subsystem
  Toggle_HallB : Subsystem
  Toggle_HallC : Subsystem
  HallStateChange : Outport
  wires:
  Mux2/1 -> HallStateChange/1
  Digital_Input_ISR_HALL_C/1 -> Toggle_HallC/Trigger
  Digital_Input_ISR_HALL_B/1 -> Toggle_HallB/Trigger
  Toggle_HallB/1(Call) -> Mux2/2
  Digital_Input_ISR_HALL_A/1 -> Toggle_HallA/Trigger
  Toggle_HallA/1(Call) -> Mux2/1
  Toggle_HallC/1(Call) -> Mux2/3

== system BLDC_OpenLoop_s32k144/S32K144 EVB/Event_Control/HallSensorInit ==
  function : TriggerPort  TriggerType=function-call  VariantControl=Variant
  Data Store Write : DataStoreWrite  DataStoreName=Hall_A_sensor
  Data Store Write1 : DataStoreWrite  DataStoreName=Hall_B_sensor
  Data Store Write2 : DataStoreWrite  DataStoreName=Hall_C_sensor
  Digital_Input_HALL_A : mbd_s32k1xx_ec_toolbox/GPIO Blocks/Digital_Input  gpio_pin=PTD11: [PTD11 | Port D I/O]  pull_resistor=None  passive_filter=off
  Digital_Input_HALL_B : mbd_s32k1xx_ec_toolbox/GPIO Blocks/Digital_Input  gpio_pin=PTD10: [PTD10 | Port D I/O]  pull_resistor=None  passive_filter=off
  Digital_Input_HALL_C : mbd_s32k1xx_ec_toolbox/GPIO Blocks/Digital_Input  gpio_pin=PTA1: [PTA1 | Port A I/O]  pull_resistor=None  passive_filter=off
  Function-Call Generator : simulink/Ports & Subsystems/Function-Call Generator  sample_time=-1  numberOfIterations=1
  Call : Outport
  wires:
  Function-Call Generator/1 -> Call/1
  Digital_Input_HALL_A/1 -> Data Store Write/1
  Digital_Input_HALL_B/1 -> Data Store Write1/1
  Digital_Input_HALL_C/1 -> Data Store Write2/1

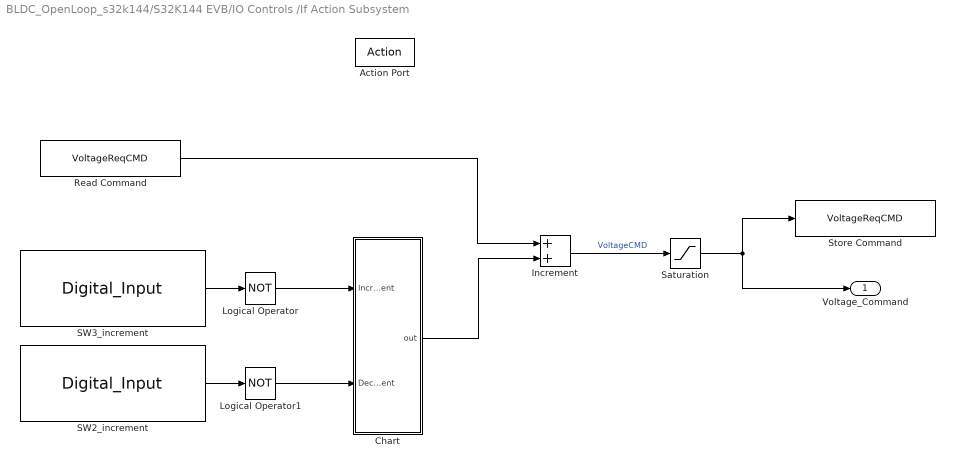
== system BLDC_OpenLoop_s32k144/S32K144 EVB/IO Controls /If Action Subsystem ==
  Action Port : ActionPort  ActionPortLabel=if((u1 == 1))
  Chart : Stateflow chart  TreatAsAtomicUnit=on
  Increment : Sum  OutMin=-12  OutMax=12  OutDataTypeStr=single
  Logical Operator : Logic  Operator=NOT  AllPortsSameDT=off  OutDataTypeStr=boolean
  Logical Operator1 : Logic  Operator=NOT  AllPortsSameDT=off  OutDataTypeStr=boolean
  Read Command : DataStoreRead  Priority=0  DataStoreName=VoltageReqCMD  DataStoreElements=VoltageReqCMD
  SW2_increment : mbd_s32k1xx_ec_toolbox/GPIO Blocks/Digital_Input  gpio_pin=PTC12: [PTC12 | Port C I/O]  pull_resistor=None  passive_filter=off
  SW3_increment : mbd_s32k1xx_ec_toolbox/GPIO Blocks/Digital_Input  gpio_pin=PTC13: [PTC13 | Port C I/O]  pull_resistor=None  passive_filter=off
  Saturation : Saturate  UpperLimit=12  LowerLimit=-12
  Store Command : DataStoreWrite  DataStoreName=VoltageReqCMD
  Voltage_Command : Outport
  wires:
  Saturation/1 -> Voltage_Command/1, Store Command/1
  Read Command/1 -> Increment/1
  Chart/1(out) -> Increment/2
  Logical Operator1/1 -> Chart/2(Decrement)
  Logical Operator/1 -> Chart/1(Increment)
  SW2_increment/1 -> Logical Operator1/1
  SW3_increment/1 -> Logical Operator/1
  Increment/1 -> Saturation/1  "VoltageCMD"

== system BLDC_OpenLoop_s32k144/S32K144 EVB/IO Controls /Subsystem ==
  START : Inport
  FAULT : Inport  Port=2
  Action Port : ActionPort  ActionPortLabel=if((u1 == 1))
  Fault : Subsystem  TreatAsAtomicUnit=on
  If : If  NumInputs=2  IfExpression=(u1 == 0) & (u2 == 0)  ElseIfExpressions=(u2 == 1)
  Ready_to_go : Subsystem  TreatAsAtomicUnit=on
  Running : Subsystem  TreatAsAtomicUnit=on
  wires:
  If/1 -> Ready_to_go/Action
  START/1 -> If/1
  If/2 -> Fault/Action
  If/3 -> Running/Action
  FAULT/1 -> If/2

== system BLDC_OpenLoop_s32k144/S32K144 EVB/Protection_Check/Subsystem ==
  In1 : Inport
  In2 : Inport  Port=2
  Action Port : ActionPort  ActionPortLabel=if((u1 == 1) & (u2 == 0))
  Check_Voltage_Current_limits : If  NumInputs=2  IfExpression=(u1 < VDC_UNDERVOLTAGE) | (u1 > VDC_OVERVOLTAGE) | (u2 > IDC_OVERCURRENT)  ShowElse=off
  FAILURE : Subsystem  TreatAsAtomicUnit=on
  wires:
  Check_Voltage_Current_limits/1 -> FAILURE/Action
  In1/1 -> Check_Voltage_Current_limits/1
  In2/1 -> Check_Voltage_Current_limits/2

== system BLDC_OpenLoop_s32k144/S32K144 EVB/Trapezoidal_Control/Commands ==
  note: 1.0    - PWM max duty cycle;
      | 12     - Vdc   max value;
  Voltage : Inport
  Abs : Abs  OutMin=0  OutMax=1  OutDataTypeStr=Inherit: Inherit via internal rule
  CCW : Constant  Value=-1  OutDataTypeStr=Inherit: Inherit via back propagation
  CW : Constant  OutDataTypeStr=Inherit: Inherit via back propagation
  Saturation : Saturate  UpperLimit=1  LowerLimit=-1
  Switch2 : Switch  OutDataTypeStr=Inherit: Inherit via back propagation
  Voltage2DutyCycle : Gain  Gain=1/12  ParamDataTypeStr=single  OutMin=-100  OutMax=100  OutDataTypeStr=single
  Direction : Outport
  PWM_Duty_Cycle : Outport  Port=2
  wires:
  Abs/1 -> PWM_Duty_Cycle/1  "DutyCycleCmd"
  Saturation/1 -> Abs/1
  CCW/1 -> Switch2/3
  Voltage/1 -> Voltage2DutyCycle/1
  CW/1 -> Switch2/1
  Voltage2DutyCycle/1 -> Saturation/1, Switch2/2
  Switch2/1 -> Direction/1

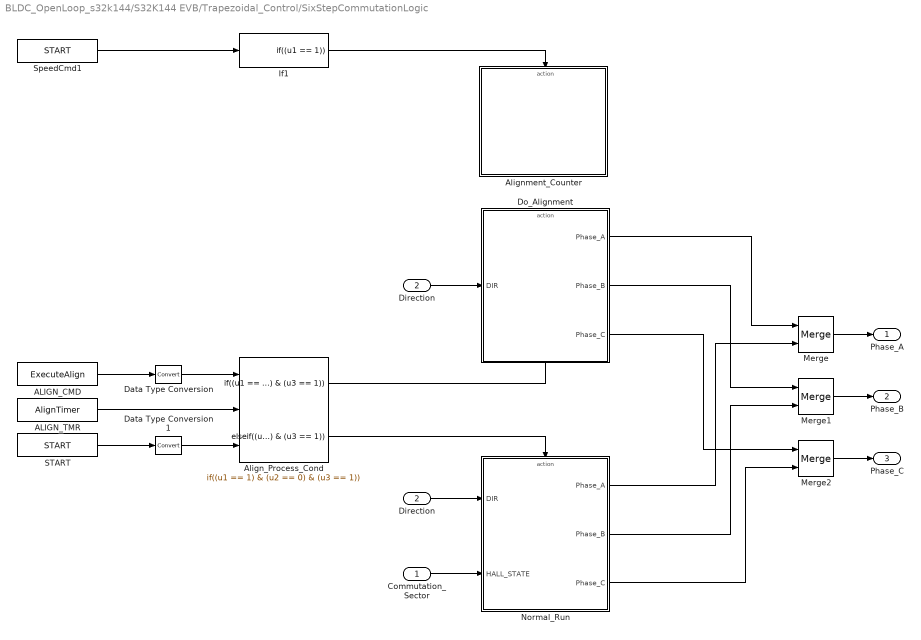
== system BLDC_OpenLoop_s32k144/S32K144 EVB/Trapezoidal_Control/SixStepCommutationLogic ==
  Commutation_Sector : Inport
  Direction : Inport  Port=2
  " ALIGN_CMD" : DataStoreRead  DataStoreName=ExecuteAlign
  " ALIGN_TMR" : DataStoreRead  DataStoreName=AlignTimer
  " START" : DataStoreRead  DataStoreName=START
  Align_Process_Cond : If  Priority=2  NumInputs=3  IfExpression=(u1 == 1) & (u2 == 0) & (u3 == 1)  ElseIfExpressions=(u1 == 0) & (u2 > 0) & (u3 == 1)  ShowElse=off
  Alignment_Counter : Subsystem
  Data Type Conversion : DataTypeConversion
  Data Type Conversion1 : DataTypeConversion
  "Direction " : InportShadow  Port=2
  Do_Alignment : Subsystem
  If1 : If  Priority=1  IfExpression=(u1 == 1)  ShowElse=off
  Merge : Merge
  Merge1 : Merge
  Merge2 : Merge
  Normal_Run : Subsystem
  SpeedCmd1 : DataStoreRead  DataStoreName=START
  Phase_A : Outport
  Phase_B : Outport  Port=2
  Phase_C : Outport  Port=3
  wires:
  Data Type Conversion/1 -> Align_Process_Cond/1
  " ALIGN_TMR"/1 -> Align_Process_Cond/2
  " ALIGN_CMD"/1 -> Data Type Conversion/1
  Commutation_Sector/1 -> Normal_Run/2(HALL_STATE)
  Direction/1 -> Normal_Run/1(DIR)
  Align_Process_Cond/2 -> Normal_Run/Action
  Align_Process_Cond/1 -> Do_Alignment/Action
  Merge/1 -> Phase_A/1
  Do_Alignment/1(Phase_A) -> Merge/1
  Normal_Run/1(Phase_A) -> Merge/2
  Do_Alignment/2(Phase_B) -> Merge1/1
  Normal_Run/2(Phase_B) -> Merge1/2
  Merge1/1 -> Phase_B/1
  Do_Alignment/3(Phase_C) -> Merge2/1
  Normal_Run/3(Phase_C) -> Merge2/2
  Merge2/1 -> Phase_C/1
  " START"/1 -> Data Type Conversion1/1
  Data Type Conversion1/1 -> Align_Process_Cond/3
  If1/1 -> Alignment_Counter/Action
  SpeedCmd1/1 -> If1/1
  "Direction "/1 -> Do_Alignment/1(DIR)

== system BLDC_OpenLoop_s32k144/S32K144 EVB/Control_Logic/enable_FTM_PDB_ADC_triggering/Custom code to reload the PDB value ==

== system BLDC_OpenLoop_s32k144/S32K144 EVB/Event_Control/ControlEventLogic/Toggle_HallA ==
  function : TriggerPort  TriggerType=function-call  VariantControl=Variant
  Data Store Read1 : DataStoreRead  DataStoreName=Hall_A_sensor
  Data Store Write1 : DataStoreWrite  DataStoreName=Hall_A_sensor
  Function-Call Generator : simulink/Ports & Subsystems/Function-Call Generator  sample_time=-1  numberOfIterations=1
  Logical Operator : Logic  Operator=NOT  AllPortsSameDT=off  OutDataTypeStr=boolean
  Call : Outport
  wires:
  Function-Call Generator/1 -> Call/1
  Data Store Read1/1 -> Logical Operator/1
  Logical Operator/1 -> Data Store Write1/1

== system BLDC_OpenLoop_s32k144/S32K144 EVB/Event_Control/ControlEventLogic/Toggle_HallB ==
  function : TriggerPort  TriggerType=function-call  VariantControl=Variant
  Data Store Read1 : DataStoreRead  DataStoreName=Hall_B_sensor
  Data Store Write1 : DataStoreWrite  DataStoreName=Hall_B_sensor
  Function-Call Generator : simulink/Ports & Subsystems/Function-Call Generator  sample_time=-1  numberOfIterations=1
  Logical Operator : Logic  Operator=NOT  AllPortsSameDT=off  OutDataTypeStr=boolean
  Call : Outport
  wires:
  Function-Call Generator/1 -> Call/1
  Data Store Read1/1 -> Logical Operator/1
  Logical Operator/1 -> Data Store Write1/1

== system BLDC_OpenLoop_s32k144/S32K144 EVB/Event_Control/ControlEventLogic/Toggle_HallC ==
  function : TriggerPort  TriggerType=function-call  VariantControl=Variant
  Data Store Read1 : DataStoreRead  DataStoreName=Hall_C_sensor
  Data Store Write1 : DataStoreWrite  DataStoreName=Hall_C_sensor
  Function-Call Generator : simulink/Ports & Subsystems/Function-Call Generator  sample_time=-1  numberOfIterations=1
  Logical Operator : Logic  Operator=NOT  AllPortsSameDT=off  OutDataTypeStr=boolean
  Call : Outport
  wires:
  Function-Call Generator/1 -> Call/1
  Data Store Read1/1 -> Logical Operator/1
  Logical Operator/1 -> Data Store Write1/1

== system BLDC_OpenLoop_s32k144/S32K144 EVB/IO Controls /Subsystem/Fault ==
  Action Port : ActionPort  ActionPortLabel=elseif((u2 == 1))
  BLUE : mbd_s32k1xx_ec_toolbox/GPIO Blocks/Digital_Output  gpio_pin=PTD0: [PTD0 | Port D I/O]  init_val=Low  drive_strength=Low
  GREEN : mbd_s32k1xx_ec_toolbox/GPIO Blocks/Digital_Output  gpio_pin=PTD16: [PTD16 | Port D I/O]  init_val=Low  drive_strength=Low
  OFF : Constant  OutDataTypeStr=boolean
  "OFF " : Constant  OutDataTypeStr=boolean
  "OFF  " : Constant  Value=0  OutDataTypeStr=boolean
  "ON " : Constant  Value=0  OutDataTypeStr=boolean
  RED : mbd_s32k1xx_ec_toolbox/GPIO Blocks/Digital_Output  gpio_pin=PTD15: [PTD15 | Port D I/O]  init_val=Low  drive_strength=Low
  "SpeedCmd " : DataStoreWrite  DataStoreName=START
  SpeedCmd 1 : DataStoreWrite  DataStoreName=READY
  wires:
  "OFF "/1 -> GREEN/1
  "ON "/1 -> RED/1
  OFF/1 -> BLUE/1
  "OFF  "/1 -> "SpeedCmd "/1, SpeedCmd 1/1

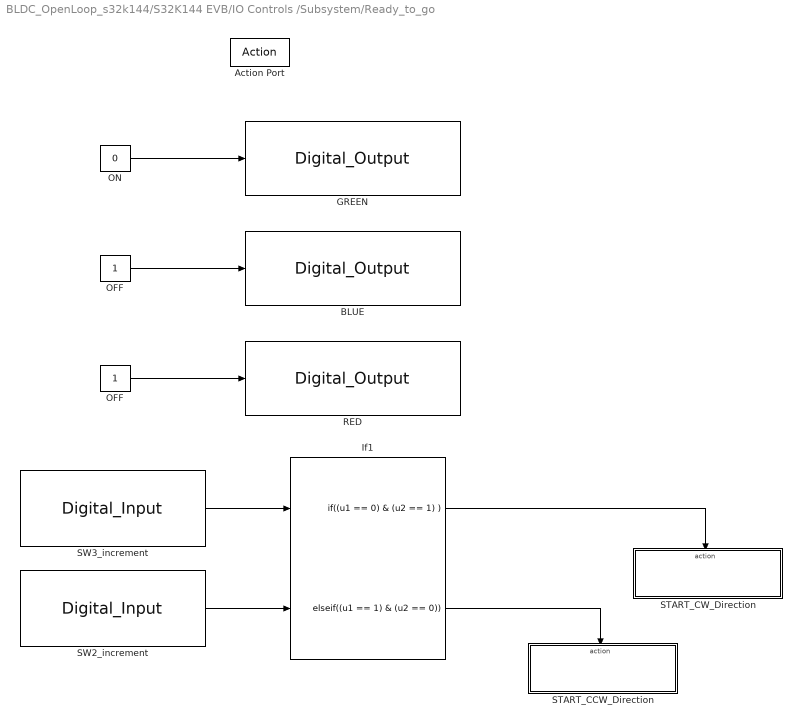
== system BLDC_OpenLoop_s32k144/S32K144 EVB/IO Controls /Subsystem/Ready_to_go ==
  Action Port : ActionPort  ActionPortLabel=if((u1 == 0) & (u2 == 0))
  BLUE : mbd_s32k1xx_ec_toolbox/GPIO Blocks/Digital_Output  gpio_pin=PTD0: [PTD0 | Port D I/O]  init_val=Low  drive_strength=Low
  GREEN : mbd_s32k1xx_ec_toolbox/GPIO Blocks/Digital_Output  gpio_pin=PTD16: [PTD16 | Port D I/O]  init_val=Low  drive_strength=Low
  If1 : If  NumInputs=2  IfExpression=(u1 == 0) & (u2 == 1)  ElseIfExpressions=(u1 == 1) & (u2 == 0)  ShowElse=off
  "OFF " : Constant  OutDataTypeStr=boolean
  "OFF  " : Constant  OutDataTypeStr=boolean
  "ON  " : Constant  Value=0  OutDataTypeStr=boolean
  RED : mbd_s32k1xx_ec_toolbox/GPIO Blocks/Digital_Output  gpio_pin=PTD15: [PTD15 | Port D I/O]  init_val=Low  drive_strength=Low
  START_CCW_Direction : Subsystem  TreatAsAtomicUnit=on
  START_CW_Direction : Subsystem  TreatAsAtomicUnit=on
  SW2_increment : mbd_s32k1xx_ec_toolbox/GPIO Blocks/Digital_Input  gpio_pin=PTC12: [PTC12 | Port C I/O]  pull_resistor=None  passive_filter=off
  SW3_increment : mbd_s32k1xx_ec_toolbox/GPIO Blocks/Digital_Input  gpio_pin=PTC13: [PTC13 | Port C I/O]  pull_resistor=None  passive_filter=off
  wires:
  "ON  "/1 -> GREEN/1
  "OFF "/1 -> RED/1
  "OFF  "/1 -> BLUE/1
  If1/1 -> START_CW_Direction/Action
  SW3_increment/1 -> If1/1
  SW2_increment/1 -> If1/2
  If1/2 -> START_CCW_Direction/Action

== system BLDC_OpenLoop_s32k144/S32K144 EVB/IO Controls /Subsystem/Running ==
  Action Port : ActionPort  ActionPortLabel=else
  BLUE : mbd_s32k1xx_ec_toolbox/GPIO Blocks/Digital_Output  gpio_pin=PTD0: [PTD0 | Port D I/O]  init_val=Low  drive_strength=Low
  GREEN : mbd_s32k1xx_ec_toolbox/GPIO Blocks/Digital_Output  gpio_pin=PTD16: [PTD16 | Port D I/O]  init_val=Low  drive_strength=Low
  "OFF " : Constant  OutDataTypeStr=boolean
  OFF_RED : Constant  OutDataTypeStr=boolean
  "ON " : Constant  Value=0  OutDataTypeStr=boolean
  RED : mbd_s32k1xx_ec_toolbox/GPIO Blocks/Digital_Output  gpio_pin=PTD15: [PTD15 | Port D I/O]  init_val=Low  drive_strength=Low
  wires:
  "OFF "/1 -> GREEN/1
  OFF_RED/1 -> RED/1
  "ON "/1 -> BLUE/1

== system BLDC_OpenLoop_s32k144/S32K144 EVB/Protection_Check/Subsystem/FAILURE ==
  Action Port : ActionPort  ActionPortLabel=if((u1 < VDC_UNDERVOLTAGE) | (u1 > VDC_OVERVOLTAGE) | (u2 > IDC_OVERCURRENT))
  FAULT_write : DataStoreWrite  DataStoreName=FAULT
  FTM_PWM_Disable_Enable : mbd_s32k1xx_ec_toolbox/Motor Control Blocks/FTM Blocks/FTM_PWM_Disable_Enable  ftmModule=3  action=Disable
  NOK : Constant  OutDataTypeStr=boolean
  TPP_Functional_Mode : mbd_msd_ec_toolbox/TPP/TPP_Functional_Mode  tppInstance=0  action=Sleep
  wires:
  NOK/1 -> FAULT_write/1

== system BLDC_OpenLoop_s32k144/S32K144 EVB/Trapezoidal_Control/SixStepCommutationLogic/Alignment_Counter ==
  Action Port : ActionPort  ActionPortLabel=if((u1 == 1))
  Align Sequence : Stateflow chart  TreatAsAtomicUnit=on
  AlignTimerIn : DataStoreRead  DataStoreName=AlignTimer
  AlignTimerOut : DataStoreWrite  DataStoreName=AlignTimer
  ExecureAlign : DataStoreWrite  DataStoreName=ExecuteAlign
  wires:
  Align Sequence/2(ExecuteAlign) -> ExecureAlign/1
  Align Sequence/1(DelayTimeOut) -> AlignTimerOut/1
  AlignTimerIn/1 -> Align Sequence/1(DelayTimeIn)

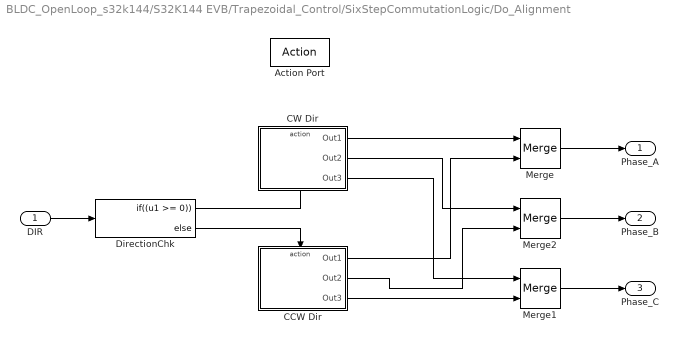
== system BLDC_OpenLoop_s32k144/S32K144 EVB/Trapezoidal_Control/SixStepCommutationLogic/Do_Alignment ==
  DIR : Inport
  Action Port : ActionPort  ActionPortLabel=if((u1 == 1) & (u2 == 0) & (u3 == 1))
  CCW Dir : Subsystem
  CW Dir : Subsystem
  DirectionChk : If  Priority=1  IfExpression=(u1 >= 0)
  Merge : Merge
  Merge1 : Merge
  Merge2 : Merge
  Phase_A : Outport
  Phase_B : Outport  Port=2
  Phase_C : Outport  Port=3
  wires:
  DIR/1 -> DirectionChk/1
  DirectionChk/1 -> CW Dir/Action
  DirectionChk/2 -> CCW Dir/Action
  Merge/1 -> Phase_A/1
  Merge1/1 -> Phase_C/1
  CCW Dir/3(Out3) -> Merge1/2
  CW Dir/3(Out3) -> Merge1/1
  CW Dir/1(Out1) -> Merge/1
  CCW Dir/1(Out1) -> Merge/2
  CW Dir/2(Out2) -> Merge2/1
  CCW Dir/2(Out2) -> Merge2/2
  Merge2/1 -> Phase_B/1

== system BLDC_OpenLoop_s32k144/S32K144 EVB/Trapezoidal_Control/SixStepCommutationLogic/Normal_Run ==
  DIR : Inport
  HALL_STATE : Inport  Port=2
  Action Port : ActionPort  ActionPortLabel=elseif((u1 == 0) & (u2 > 0) & (u3 == 1))
  CommutationTableLookup : Stateflow chart  TreatAsAtomicUnit=on
  Phase_A : Outport
  Phase_B : Outport  Port=2
  Phase_C : Outport  Port=3
  wires:
  CommutationTableLookup/2(Phase_B) -> Phase_B/1
  DIR/1 -> CommutationTableLookup/2(DIR)
  HALL_STATE/1 -> CommutationTableLookup/1(HALL_STATE)
  CommutationTableLookup/3(Phase_C) -> Phase_C/1
  CommutationTableLookup/1(Phase_A) -> Phase_A/1

== system BLDC_OpenLoop_s32k144/S32K144 EVB/IO Controls /Subsystem/Ready_to_go/START_CCW_Direction ==
  Action Port : ActionPort  ActionPortLabel=elseif((u1 == 1) & (u2 == 0) )
  Constant : Constant  Value=-V0  OutDataTypeStr=single
  ON : Constant  OutDataTypeStr=boolean
  "SpeedCmd " : DataStoreWrite  DataStoreName=START
  Store Command : DataStoreWrite  DataStoreName=VoltageReqCMD
  wires:
  Constant/1 -> Store Command/1
  ON/1 -> "SpeedCmd "/1

== system BLDC_OpenLoop_s32k144/S32K144 EVB/IO Controls /Subsystem/Ready_to_go/START_CW_Direction ==
  Action Port : ActionPort  ActionPortLabel=if((u1 == 0) & (u2 == 1) )
  Constant : Constant  Value=V0  OutDataTypeStr=single
  ON : Constant  OutDataTypeStr=boolean
  "SpeedCmd " : DataStoreWrite  DataStoreName=START
  Store Command : DataStoreWrite  DataStoreName=VoltageReqCMD
  wires:
  ON/1 -> "SpeedCmd "/1
  Constant/1 -> Store Command/1

== system BLDC_OpenLoop_s32k144/S32K144 EVB/Trapezoidal_Control/SixStepCommutationLogic/Do_Alignment/CCW Dir ==
  Action Port : ActionPort  ActionPortLabel=else
  Constant : Constant  OutDataTypeStr=Inherit: Inherit via back propagation
  Constant1 : Constant  Value=0  OutDataTypeStr=Inherit: Inherit via back propagation
  Constant2 : Constant  Value=2  OutDataTypeStr=Inherit: Inherit via back propagation
  Out1 : Outport
  Out2 : Outport  Port=2
  Out3 : Outport  Port=3
  wires:
  Constant1/1 -> Out2/1
  Constant2/1 -> Out3/1
  Constant/1 -> Out1/1
